simulink model "tank"  (R2015b)
settings: Solver=FixedStepDiscrete  StartTime=0.0  StopTime=inf  FixedStep=1e-3  RelTol=1e-3
libraries: sh_lib x74, nesl_utility x46, fl_lib x40, dspnetwork x33
(part 2 of 3)

== system tank/Virtual Gas Pipeline /The Gas Pipeline/Ball Valve2 ==
  Relief Valve Control : Inport
  Ball Valve : sh_lib/Valves/Flow Control Valves/Ball Valve  d_ball=8 in  d_orif=6 in  x_0=0 m  C_d=0.65  Re_cr=10  A_leak=1e-12 m^2
  Simulink-PS Converter : nesl_utility/Simulink-PS Converter  PhysicalDomain=network_engine_domain  SubClassName=ps_input  LeftPortType=input  RightPortType=output  PseudoPeriodic=off  Frequencies=[]  NoiseDistribution=none  NoiseParameters=[]  Unit=1  AffineConversion=off  InputFiltering=off  SimscapeFilterOrder=1  InputFilterTimeConstant=0.001  UdotUserProvided=1
  Inlet : PMIOPort  Port=1  Side=Left
  outlet : PMIOPort  Port=2  Side=Right
  wires:
  Relief Valve Control/1 -> Simulink-PS Converter/1
  connections:
  Simulink-PS Converter/RConn1 -- Ball Valve/LConn1
  Inlet/RConn1 -- Ball Valve/LConn2
  outlet/RConn1 -- Ball Valve/RConn1

== system tank/Virtual Gas Pipeline /The Gas Pipeline/Ball Valve3 ==
  Relief Valve Control : Inport
  Ball Valve : sh_lib/Valves/Flow Control Valves/Ball Valve  d_ball=8 in  d_orif=6 in  x_0=0 m  C_d=0.65  Re_cr=10  A_leak=1e-12 m^2
  Simulink-PS Converter : nesl_utility/Simulink-PS Converter  PhysicalDomain=network_engine_domain  SubClassName=ps_input  LeftPortType=input  RightPortType=output  PseudoPeriodic=off  Frequencies=[]  NoiseDistribution=none  NoiseParameters=[]  Unit=1  AffineConversion=off  InputFiltering=off  SimscapeFilterOrder=1  InputFilterTimeConstant=0.001  UdotUserProvided=1
  Inlet : PMIOPort  Port=1  Side=Left
  outlet : PMIOPort  Port=2  Side=Right
  wires:
  Relief Valve Control/1 -> Simulink-PS Converter/1
  connections:
  Simulink-PS Converter/RConn1 -- Ball Valve/LConn1
  Inlet/RConn1 -- Ball Valve/LConn2
  outlet/RConn1 -- Ball Valve/RConn1

== system tank/Virtual Gas Pipeline /The Gas Pipeline/Ball Valve4 ==
  valve : Inport
  Ball Valve : sh_lib/Valves/Flow Control Valves/Ball Valve  d_ball=18 in  d_orif=16 in  x_0=0 m  C_d=0.65  Re_cr=10  A_leak=1e-12 m^2
  Simulink-PS Converter : nesl_utility/Simulink-PS Converter  PhysicalDomain=network_engine_domain  SubClassName=ps_input  LeftPortType=input  RightPortType=output  PseudoPeriodic=off  Frequencies=[]  NoiseDistribution=none  NoiseParameters=[]  Unit=1  AffineConversion=off  InputFiltering=off  SimscapeFilterOrder=1  InputFilterTimeConstant=0.001  UdotUserProvided=1
  Inlet : PMIOPort  Port=1  Side=Left
  outlet : PMIOPort  Port=2  Side=Right
  wires:
  valve/1 -> Simulink-PS Converter/1
  connections:
  Simulink-PS Converter/RConn1 -- Ball Valve/LConn1
  Inlet/RConn1 -- Ball Valve/LConn2
  outlet/RConn1 -- Ball Valve/RConn1

== system tank/Virtual Gas Pipeline /The Gas Pipeline/Ball Valve5 ==
  valve : Inport
  Ball Valve : sh_lib/Valves/Flow Control Valves/Ball Valve  d_ball=18 in  d_orif=16 in  x_0=0 m  C_d=0.65  Re_cr=10  A_leak=1e-12 m^2
  Simulink-PS Converter : nesl_utility/Simulink-PS Converter  PhysicalDomain=network_engine_domain  SubClassName=ps_input  LeftPortType=input  RightPortType=output  PseudoPeriodic=off  Frequencies=[]  NoiseDistribution=none  NoiseParameters=[]  Unit=1  AffineConversion=off  InputFiltering=off  SimscapeFilterOrder=1  InputFilterTimeConstant=0.001  UdotUserProvided=1
  Inlet : PMIOPort  Port=1  Side=Left
  outlet : PMIOPort  Port=2  Side=Right
  wires:
  valve/1 -> Simulink-PS Converter/1
  connections:
  Simulink-PS Converter/RConn1 -- Ball Valve/LConn1
  Inlet/RConn1 -- Ball Valve/LConn2
  outlet/RConn1 -- Ball Valve/RConn1

== system tank/Virtual Gas Pipeline /The Gas Pipeline/Ball Valve6 ==
  valve : Inport
  Ball Valve : sh_lib/Valves/Flow Control Valves/Ball Valve  d_ball=8 in  d_orif=6 in  x_0=0 m  C_d=0.65  Re_cr=10  A_leak=1e-12 m^2
  Simulink-PS Converter : nesl_utility/Simulink-PS Converter  PhysicalDomain=network_engine_domain  SubClassName=ps_input  LeftPortType=input  RightPortType=output  PseudoPeriodic=off  Frequencies=[]  NoiseDistribution=none  NoiseParameters=[]  Unit=1  AffineConversion=off  InputFiltering=off  SimscapeFilterOrder=1  InputFilterTimeConstant=0.001  UdotUserProvided=1
  Inlet : PMIOPort  Port=1  Side=Left
  outlet : PMIOPort  Port=2  Side=Right
  wires:
  valve/1 -> Simulink-PS Converter/1
  connections:
  Simulink-PS Converter/RConn1 -- Ball Valve/LConn1
  Inlet/RConn1 -- Ball Valve/LConn2
  outlet/RConn1 -- Ball Valve/RConn1

== system tank/Virtual Gas Pipeline /The Gas Pipeline/Ball Valve7 ==
  valve : Inport
  Ball Valve : sh_lib/Valves/Flow Control Valves/Ball Valve  d_ball=8 in  d_orif=6 in  x_0=0 m  C_d=0.65  Re_cr=10  A_leak=1e-12 m^2
  Simulink-PS Converter : nesl_utility/Simulink-PS Converter  PhysicalDomain=network_engine_domain  SubClassName=ps_input  LeftPortType=input  RightPortType=output  PseudoPeriodic=off  Frequencies=[]  NoiseDistribution=none  NoiseParameters=[]  Unit=1  AffineConversion=off  InputFiltering=off  SimscapeFilterOrder=1  InputFilterTimeConstant=0.001  UdotUserProvided=1
  Inlet : PMIOPort  Port=1  Side=Left
  outlet : PMIOPort  Port=2  Side=Right
  wires:
  valve/1 -> Simulink-PS Converter/1
  connections:
  Simulink-PS Converter/RConn1 -- Ball Valve/LConn1
  Inlet/RConn1 -- Ball Valve/LConn2
  outlet/RConn1 -- Ball Valve/RConn1

== system tank/Virtual Gas Pipeline /The Gas Pipeline/Flow Measurement (KL//Hr) ==
  Constant : Constant  Value=3600
  Hydraulic Flow Rate Sensor : fl_lib/Hydraulic/Hydraulic Sensors/Hydraulic Flow Rate Sensor
  PS-Simulink Converter3 : nesl_utility/PS-Simulink Converter  PhysicalDomain=network_engine_domain  SubClassName=ps_output  LeftPortType=input  RightPortType=output  PseudoPeriodic=off  Frequencies=[]  Unit=m^3/s  AffineConversion=off
  Product : Product
  Inlet reference : PMIOPort  Port=1  Side=Left
  " Outlet Reference" : PMIOPort  Port=2  Side=Left
  Display out : Outport
  wires:
  Product/1 -> Display out/1
  Constant/1 -> Product/2
  PS-Simulink Converter3/1 -> Product/1
  connections:
  PS-Simulink Converter3/LConn1 -- Hydraulic Flow Rate Sensor/RConn1
  Hydraulic Flow Rate Sensor/RConn2 -- " Outlet Reference"/RConn1
  Hydraulic Flow Rate Sensor/LConn1 -- Inlet reference/RConn1

== system tank/Virtual Gas Pipeline /The Gas Pipeline/Flow Measurement (KL//Hr)1 ==
  Constant : Constant  Value=3600
  Hydraulic Flow Rate Sensor : fl_lib/Hydraulic/Hydraulic Sensors/Hydraulic Flow Rate Sensor
  PS-Simulink Converter3 : nesl_utility/PS-Simulink Converter  PhysicalDomain=network_engine_domain  SubClassName=ps_output  LeftPortType=input  RightPortType=output  PseudoPeriodic=off  Frequencies=[]  Unit=m^3/s  AffineConversion=off
  Product : Product
  Inlet reference : PMIOPort  Port=1  Side=Left
  " Outlet Reference" : PMIOPort  Port=2  Side=Left
  Display out : Outport
  wires:
  Product/1 -> Display out/1
  Constant/1 -> Product/2
  PS-Simulink Converter3/1 -> Product/1
  connections:
  PS-Simulink Converter3/LConn1 -- Hydraulic Flow Rate Sensor/RConn1
  Hydraulic Flow Rate Sensor/RConn2 -- " Outlet Reference"/RConn1
  Hydraulic Flow Rate Sensor/LConn1 -- Inlet reference/RConn1

== system tank/Virtual Gas Pipeline /The Gas Pipeline/Flow Measurement (KL//Hr)2 ==
  Constant : Constant  Value=3600
  Hydraulic Flow Rate Sensor : fl_lib/Hydraulic/Hydraulic Sensors/Hydraulic Flow Rate Sensor
  PS-Simulink Converter3 : nesl_utility/PS-Simulink Converter  PhysicalDomain=network_engine_domain  SubClassName=ps_output  LeftPortType=input  RightPortType=output  PseudoPeriodic=off  Frequencies=[]  Unit=m^3/s  AffineConversion=off
  Product : Product
  Inlet reference : PMIOPort  Port=1  Side=Left
  " Outlet Reference" : PMIOPort  Port=2  Side=Left
  Display out : Outport
  wires:
  Product/1 -> Display out/1
  Constant/1 -> Product/2
  PS-Simulink Converter3/1 -> Product/1
  connections:
  PS-Simulink Converter3/LConn1 -- Hydraulic Flow Rate Sensor/RConn1
  Hydraulic Flow Rate Sensor/RConn2 -- " Outlet Reference"/RConn1
  Hydraulic Flow Rate Sensor/LConn1 -- Inlet reference/RConn1

== system tank/Virtual Gas Pipeline /The Gas Pipeline/Flow Measurement (KL//Hr)3 ==
  Constant : Constant  Value=3600
  Hydraulic Flow Rate Sensor : fl_lib/Hydraulic/Hydraulic Sensors/Hydraulic Flow Rate Sensor
  PS-Simulink Converter3 : nesl_utility/PS-Simulink Converter  PhysicalDomain=network_engine_domain  SubClassName=ps_output  LeftPortType=input  RightPortType=output  PseudoPeriodic=off  Frequencies=[]  Unit=m^3/s  AffineConversion=off
  Product : Product
  Inlet reference : PMIOPort  Port=1  Side=Left
  " Outlet Reference" : PMIOPort  Port=2  Side=Left
  Display out : Outport
  wires:
  Product/1 -> Display out/1
  Constant/1 -> Product/2
  PS-Simulink Converter3/1 -> Product/1
  connections:
  PS-Simulink Converter3/LConn1 -- Hydraulic Flow Rate Sensor/RConn1
  Hydraulic Flow Rate Sensor/RConn2 -- " Outlet Reference"/RConn1
  Hydraulic Flow Rate Sensor/LConn1 -- Inlet reference/RConn1

== system tank/Virtual Gas Pipeline /The Gas Pipeline/Flow Measurement (KL//Hr)4 ==
  Constant : Constant  Value=3600
  Hydraulic Flow Rate Sensor : fl_lib/Hydraulic/Hydraulic Sensors/Hydraulic Flow Rate Sensor
  PS-Simulink Converter3 : nesl_utility/PS-Simulink Converter  PhysicalDomain=network_engine_domain  SubClassName=ps_output  LeftPortType=input  RightPortType=output  PseudoPeriodic=off  Frequencies=[]  Unit=m^3/s  AffineConversion=off
  Product : Product
  Inlet reference : PMIOPort  Port=1  Side=Left
  " Outlet Reference" : PMIOPort  Port=2  Side=Left
  Display out : Outport
  wires:
  Product/1 -> Display out/1
  Constant/1 -> Product/2
  PS-Simulink Converter3/1 -> Product/1
  connections:
  PS-Simulink Converter3/LConn1 -- Hydraulic Flow Rate Sensor/RConn1
  Hydraulic Flow Rate Sensor/RConn2 -- " Outlet Reference"/RConn1
  Hydraulic Flow Rate Sensor/LConn1 -- Inlet reference/RConn1

== system tank/Virtual Gas Pipeline /The Gas Pipeline/Flow Measurement (KL//Hr)5 ==
  Constant : Constant  Value=3600
  Hydraulic Flow Rate Sensor : fl_lib/Hydraulic/Hydraulic Sensors/Hydraulic Flow Rate Sensor
  PS-Simulink Converter3 : nesl_utility/PS-Simulink Converter  PhysicalDomain=network_engine_domain  SubClassName=ps_output  LeftPortType=input  RightPortType=output  PseudoPeriodic=off  Frequencies=[]  Unit=m^3/s  AffineConversion=off
  Product : Product
  Inlet reference : PMIOPort  Port=1  Side=Left
  " Outlet Reference" : PMIOPort  Port=2  Side=Left
  Display out : Outport
  wires:
  Product/1 -> Display out/1
  Constant/1 -> Product/2
  PS-Simulink Converter3/1 -> Product/1
  connections:
  PS-Simulink Converter3/LConn1 -- Hydraulic Flow Rate Sensor/RConn1
  Hydraulic Flow Rate Sensor/RConn2 -- " Outlet Reference"/RConn1
  Hydraulic Flow Rate Sensor/LConn1 -- Inlet reference/RConn1

== system tank/Virtual Gas Pipeline /The Gas Pipeline/Flow Measurement (KL//Hr)6 ==
  Constant : Constant  Value=3600
  Hydraulic Flow Rate Sensor : fl_lib/Hydraulic/Hydraulic Sensors/Hydraulic Flow Rate Sensor
  PS-Simulink Converter3 : nesl_utility/PS-Simulink Converter  PhysicalDomain=network_engine_domain  SubClassName=ps_output  LeftPortType=input  RightPortType=output  PseudoPeriodic=off  Frequencies=[]  Unit=m^3/s  AffineConversion=off
  Product : Product
  Inlet reference : PMIOPort  Port=1  Side=Left
  " Outlet Reference" : PMIOPort  Port=2  Side=Left
  Display out : Outport
  wires:
  Product/1 -> Display out/1
  Constant/1 -> Product/2
  PS-Simulink Converter3/1 -> Product/1
  connections:
  PS-Simulink Converter3/LConn1 -- Hydraulic Flow Rate Sensor/RConn1
  Hydraulic Flow Rate Sensor/RConn2 -- " Outlet Reference"/RConn1
  Hydraulic Flow Rate Sensor/LConn1 -- Inlet reference/RConn1

== system tank/Virtual Gas Pipeline /The Gas Pipeline/Flow Measurement (KL//Hr)7 ==
  Constant : Constant  Value=3600
  Hydraulic Flow Rate Sensor : fl_lib/Hydraulic/Hydraulic Sensors/Hydraulic Flow Rate Sensor
  PS-Simulink Converter3 : nesl_utility/PS-Simulink Converter  PhysicalDomain=network_engine_domain  SubClassName=ps_output  LeftPortType=input  RightPortType=output  PseudoPeriodic=off  Frequencies=[]  Unit=m^3/s  AffineConversion=off
  Product : Product
  Inlet reference : PMIOPort  Port=1  Side=Left
  " Outlet Reference" : PMIOPort  Port=2  Side=Left
  Display out : Outport
  wires:
  Product/1 -> Display out/1
  Constant/1 -> Product/2
  PS-Simulink Converter3/1 -> Product/1
  connections:
  PS-Simulink Converter3/LConn1 -- Hydraulic Flow Rate Sensor/RConn1
  Hydraulic Flow Rate Sensor/RConn2 -- " Outlet Reference"/RConn1
  Hydraulic Flow Rate Sensor/LConn1 -- Inlet reference/RConn1

== system tank/Virtual Gas Pipeline /The Gas Pipeline/Pressure Sensor ==
  Hydraulic Reference3 : fl_lib/Hydraulic/Hydraulic Elements/Hydraulic Reference
  Ideal Hydraulic Pressure Sensor3 : fl_lib/Hydraulic/Hydraulic Sensors/Hydraulic Pressure Sensor
  PS-Simulink Converter3 : nesl_utility/PS-Simulink Converter  PhysicalDomain=network_engine_domain  SubClassName=ps_output  LeftPortType=input  RightPortType=output  PseudoPeriodic=off  Frequencies=[]  Unit=Pa  AffineConversion=off
  Point : PMIOPort  Port=1  Side=Left
  " Display" : Outport
  wires:
  PS-Simulink Converter3/1 -> " Display"/1
  connections:
  Point/RConn1 -- Ideal Hydraulic Pressure Sensor3/LConn1
  Ideal Hydraulic Pressure Sensor3/RConn1 -- Hydraulic Reference3/LConn1
  Ideal Hydraulic Pressure Sensor3/RConn2 -- PS-Simulink Converter3/LConn1

== system tank/Virtual Gas Pipeline /The Gas Pipeline/Pressure Sensor1 ==
  Hydraulic Reference3 : fl_lib/Hydraulic/Hydraulic Elements/Hydraulic Reference
  Ideal Hydraulic Pressure Sensor3 : fl_lib/Hydraulic/Hydraulic Sensors/Hydraulic Pressure Sensor
  PS-Simulink Converter3 : nesl_utility/PS-Simulink Converter  PhysicalDomain=network_engine_domain  SubClassName=ps_output  LeftPortType=input  RightPortType=output  PseudoPeriodic=off  Frequencies=[]  Unit=Pa  AffineConversion=off
  Point : PMIOPort  Port=1  Side=Left
  " Display" : Outport
  wires:
  PS-Simulink Converter3/1 -> " Display"/1
  connections:
  Point/RConn1 -- Ideal Hydraulic Pressure Sensor3/LConn1
  Ideal Hydraulic Pressure Sensor3/RConn1 -- Hydraulic Reference3/LConn1
  Ideal Hydraulic Pressure Sensor3/RConn2 -- PS-Simulink Converter3/LConn1

== system tank/Virtual Gas Pipeline /The Gas Pipeline/Pressure Sensor2 ==
  Hydraulic Reference3 : fl_lib/Hydraulic/Hydraulic Elements/Hydraulic Reference
  Ideal Hydraulic Pressure Sensor3 : fl_lib/Hydraulic/Hydraulic Sensors/Hydraulic Pressure Sensor
  PS-Simulink Converter3 : nesl_utility/PS-Simulink Converter  PhysicalDomain=network_engine_domain  SubClassName=ps_output  LeftPortType=input  RightPortType=output  PseudoPeriodic=off  Frequencies=[]  Unit=Pa  AffineConversion=off
  Point : PMIOPort  Port=1  Side=Left
  " Display" : Outport
  wires:
  PS-Simulink Converter3/1 -> " Display"/1
  connections:
  Point/RConn1 -- Ideal Hydraulic Pressure Sensor3/LConn1
  Ideal Hydraulic Pressure Sensor3/RConn1 -- Hydraulic Reference3/LConn1
  Ideal Hydraulic Pressure Sensor3/RConn2 -- PS-Simulink Converter3/LConn1

== system tank/Virtual Gas Pipeline /The Gas Pipeline/Pressure Sensor3 ==
  Hydraulic Reference3 : fl_lib/Hydraulic/Hydraulic Elements/Hydraulic Reference
  Ideal Hydraulic Pressure Sensor3 : fl_lib/Hydraulic/Hydraulic Sensors/Hydraulic Pressure Sensor
  PS-Simulink Converter3 : nesl_utility/PS-Simulink Converter  PhysicalDomain=network_engine_domain  SubClassName=ps_output  LeftPortType=input  RightPortType=output  PseudoPeriodic=off  Frequencies=[]  Unit=Pa  AffineConversion=off
  Point : PMIOPort  Port=1  Side=Left
  " Display" : Outport
  wires:
  PS-Simulink Converter3/1 -> " Display"/1
  connections:
  Point/RConn1 -- Ideal Hydraulic Pressure Sensor3/LConn1
  Ideal Hydraulic Pressure Sensor3/RConn1 -- Hydraulic Reference3/LConn1
  Ideal Hydraulic Pressure Sensor3/RConn2 -- PS-Simulink Converter3/LConn1

== system tank/Virtual Gas Pipeline /The Gas Pipeline/Pressure Sensor4 ==
  Hydraulic Reference3 : fl_lib/Hydraulic/Hydraulic Elements/Hydraulic Reference
  Ideal Hydraulic Pressure Sensor3 : fl_lib/Hydraulic/Hydraulic Sensors/Hydraulic Pressure Sensor
  PS-Simulink Converter3 : nesl_utility/PS-Simulink Converter  PhysicalDomain=network_engine_domain  SubClassName=ps_output  LeftPortType=input  RightPortType=output  PseudoPeriodic=off  Frequencies=[]  Unit=Pa  AffineConversion=off
  Point : PMIOPort  Port=1  Side=Left
  " Display" : Outport
  wires:
  PS-Simulink Converter3/1 -> " Display"/1
  connections:
  Point/RConn1 -- Ideal Hydraulic Pressure Sensor3/LConn1
  Ideal Hydraulic Pressure Sensor3/RConn1 -- Hydraulic Reference3/LConn1
  Ideal Hydraulic Pressure Sensor3/RConn2 -- PS-Simulink Converter3/LConn1

== system tank/Virtual Gas Pipeline /The Gas Pipeline/Primary Pumping station (500 kl//hr) ==
  Pump 1 Control : Inport
  Fixed-Displacement Pump : sh_lib/Pumps and Motors/Fixed-Displacement Pump  D=.0027777777 m^3/rev  efficiency_vol=0.92  efficiency_tot=0.8  pr_nominal=8.5 bar  w_nominal=3000 rpm  visc_nominal=18 cSt  dens_nominal=900 kg/m^3  k_leak=1e-11 m^3/s/Pa  efficiency_mech=0.7
  Ideal Angular Velocity Source : fl_lib/Mechanical/Mechanical Sources/Ideal Angular Velocity Source
  Mechanical Rotational Reference : fl_lib/Mechanical/Rotational Elements/Mechanical Rotational Reference
  Simulink-PS Converter : nesl_utility/Simulink-PS Converter  PhysicalDomain=network_engine_domain  SubClassName=ps_input  LeftPortType=input  RightPortType=output  PseudoPeriodic=off  Frequencies=[]  NoiseDistribution=none  NoiseParameters=[]  Unit=1  AffineConversion=off  InputFiltering=off  SimscapeFilterOrder=1  InputFilterTimeConstant=0.001  UdotUserProvided=1
  Solver Configuration : nesl_utility/Solver Configuration  PhysicalDomain=network_engine_domain  SubClassName=solver  LeftPortType=input  RightPortType=generic  Accelerate=off  Tones=[]  Harmonics=[]  SimulateNoise=off  Profile=off  UseLocalSampling=off  EnableSwitchedLinearOptims=on  FrequencyDomain=off  UseCCode=off  RelTol=0.001  AbsTol=1e-06  MinStep=1e-09  ToWorkspace=off  RevertToSquareIcSolve=off  NumHomotopyIterations=100  PhasorMode=off  PhasorModeNumHarmonics=1  DoDC=on  ResidualTolerance=1  UseLocalSolver=on  LocalSolverChoice=NE_TRAPEZOIDAL_ADVANCER  LocalSolverSampleTime=0.001  DoFixedCost=on  MaxNonlinIter=12  MaxModeIter=2  LinearAlgebra=Full  DelaysMemoryBudget=1024  AutomaticFiltering=on  FilteringTimeConstant=0.001
  Switch1 : Switch  Threshold=1
  rpm : Constant  Value=3000
  rpm1 : Constant  Value=0
  Pump Outlet : PMIOPort  Port=1  Side=Right
  Pump Inlet : PMIOPort  Port=2  Side=Left
  wires:
  Pump 1 Control/1 -> Switch1/2
  rpm1/1 -> Switch1/3
  Switch1/1 -> Simulink-PS Converter/1
  rpm/1 -> Switch1/1
  connections:
  Mechanical Rotational Reference/LConn1 -- Ideal Angular Velocity Source/RConn2
  Simulink-PS Converter/RConn1 -- Ideal Angular Velocity Source/RConn1
  Pump Outlet/RConn1 -- Fixed-Displacement Pump/RConn1
  Fixed-Displacement Pump/LConn1 -- Solver Configuration/RConn1 -- Ideal Angular Velocity Source/LConn1
  Pump Inlet/RConn1 -- Fixed-Displacement Pump/RConn2

== system tank/Virtual Gas Pipeline /The Gas Pipeline/Recirculation valve ==
  valve : Inport
  Ball Valve : sh_lib/Valves/Flow Control Valves/Ball Valve  d_ball=18 in  d_orif=16 in  x_0=0 m  C_d=0.65  Re_cr=10  A_leak=1e-12 m^2
  Simulink-PS Converter : nesl_utility/Simulink-PS Converter  PhysicalDomain=network_engine_domain  SubClassName=ps_input  LeftPortType=input  RightPortType=output  PseudoPeriodic=off  Frequencies=[]  NoiseDistribution=none  NoiseParameters=[]  Unit=1  AffineConversion=off  InputFiltering=off  SimscapeFilterOrder=1  InputFilterTimeConstant=0.001  UdotUserProvided=1
  Inlet : PMIOPort  Port=1  Side=Left
  outlet : PMIOPort  Port=2  Side=Right
  wires:
  valve/1 -> Simulink-PS Converter/1
  connections:
  Simulink-PS Converter/RConn1 -- Ball Valve/LConn1
  Inlet/RConn1 -- Ball Valve/LConn2
  outlet/RConn1 -- Ball Valve/RConn1

== system tank/Virtual Gas Pipeline /The Gas Pipeline/Relief Valve 1  ==
  Relief Valve 1 Control : Inport
  Relief Valve 1 : sh_lib/Valves/Flow Control Valves/Ball Valve  d_ball=10 in  d_orif=8 in  x_0=0 m  C_d=0.65  Re_cr=10  A_leak=1e-12 m^2
  Simulink-PS Converter1 : nesl_utility/Simulink-PS Converter  PhysicalDomain=network_engine_domain  SubClassName=ps_input  LeftPortType=input  RightPortType=output  PseudoPeriodic=off  Frequencies=[]  NoiseDistribution=none  NoiseParameters=[]  Unit=1  AffineConversion=off  InputFiltering=off  SimscapeFilterOrder=1  InputFilterTimeConstant=0.001  UdotUserProvided=1
  Inlet : PMIOPort  Port=1  Side=Left
  Outlet : PMIOPort  Port=2  Side=Left
  wires:
  Relief Valve 1 Control/1 -> Simulink-PS Converter1/1
  connections:
  Outlet/RConn1 -- Relief Valve 1/RConn1
  Simulink-PS Converter1/RConn1 -- Relief Valve 1/LConn1
  Inlet/RConn1 -- Relief Valve 1/LConn2

== system tank/Virtual Gas Pipeline /The Gas Pipeline/Return line ==
  Hydraulic Pipeline4 : sh_lib/Pipelines/Hydraulic Pipeline  cs_type=1  d_in=16 in  area=1e-04 m^2  D_h=0.0112 m  s_factor=64  length=3000 m  length_ad=200 m  roughness=1.5e-05 m  Re_lam=2e+03  Re_turb=4e+03  wall_type=1  pr_r_coef=2e-12 m/Pa  time_const=0.01 s  k_sh=1.4  initial_pressure=0 Pa
  Sudden Area Change1 : sh_lib/Local Hydraulic Resistances/Sudden Area Change  small_diam=8 in  large_diam=16 in  mdl_type=1  kp_c=1  Re_vec="[  -4e+03 -3e+03 -2e+03 -1000 -500 -200 -100 -50 -40 -30 -20 -15 -10 10 20 30 40 50 100 200 500 1000 2e+03 4e+03 5e+03 1e+04 ]"  loss_coeff_vec="[  0.25 0.3 0.65 0.9 0.65 0.75 0.9 1.15 1.35 1.65 2.3 2.8 3.1 5 2.7 1.8 1.46 1.3 0.9 0.65 0.42 0.3 0.2 0.4 0.42 0.25 ]"  interp_method=2  extrap_method=2  Re_cr=110
  Return Inlet : PMIOPort  Port=1  Side=Left
  Return Outlet : PMIOPort  Port=2  Side=Right
  connections:
  Sudden Area Change1/RConn1 -- Hydraulic Pipeline4/LConn1
  Return Inlet/RConn1 -- Sudden Area Change1/LConn1
  Return Outlet/RConn1 -- Hydraulic Pipeline4/RConn1

== system tank/Virtual Gas Pipeline /The Gas Pipeline/Return line 1  ==
  Hydraulic Pipeline4 : sh_lib/Pipelines/Hydraulic Pipeline  cs_type=1  d_in=16 in  area=1e-04 m^2  D_h=0.0112 m  s_factor=64  length=3000 m  length_ad=200 m  roughness=1.5e-05 m  Re_lam=2e+03  Re_turb=4e+03  wall_type=1  pr_r_coef=2e-12 m/Pa  time_const=0.01 s  k_sh=1.4  initial_pressure=0 Pa
  Sudden Area Change1 : sh_lib/Local Hydraulic Resistances/Sudden Area Change  small_diam=8 in  large_diam=16 in  mdl_type=1  kp_c=1  Re_vec="[  -4e+03 -3e+03 -2e+03 -1000 -500 -200 -100 -50 -40 -30 -20 -15 -10 10 20 30 40 50 100 200 500 1000 2e+03 4e+03 5e+03 1e+04 ]"  loss_coeff_vec="[  0.25 0.3 0.65 0.9 0.65 0.75 0.9 1.15 1.35 1.65 2.3 2.8 3.1 5 2.7 1.8 1.46 1.3 0.9 0.65 0.42 0.3 0.2 0.4 0.42 0.25 ]"  interp_method=2  extrap_method=2  Re_cr=110
  Return Inlet : PMIOPort  Port=1  Side=Left
  Return Outlet : PMIOPort  Port=2  Side=Right
  connections:
  Sudden Area Change1/RConn1 -- Hydraulic Pipeline4/LConn1
  Return Inlet/RConn1 -- Sudden Area Change1/LConn1
  Return Outlet/RConn1 -- Hydraulic Pipeline4/RConn1

== system tank/Virtual Gas Pipeline /The Gas Pipeline/Return line1 ==
  Hydraulic Pipeline4 : sh_lib/Pipelines/Hydraulic Pipeline  cs_type=1  d_in=16 in  area=1e-04 m^2  D_h=0.0112 m  s_factor=64  length=3000 m  length_ad=200 m  roughness=1.5e-05 m  Re_lam=2e+03  Re_turb=4e+03  wall_type=1  pr_r_coef=2e-12 m/Pa  time_const=0.01 s  k_sh=1.4  initial_pressure=0 Pa
  Sudden Area Change1 : sh_lib/Local Hydraulic Resistances/Sudden Area Change  small_diam=8 in  large_diam=16 in  mdl_type=1  kp_c=1  Re_vec="[  -4e+03 -3e+03 -2e+03 -1000 -500 -200 -100 -50 -40 -30 -20 -15 -10 10 20 30 40 50 100 200 500 1000 2e+03 4e+03 5e+03 1e+04 ]"  loss_coeff_vec="[  0.25 0.3 0.65 0.9 0.65 0.75 0.9 1.15 1.35 1.65 2.3 2.8 3.1 5 2.7 1.8 1.46 1.3 0.9 0.65 0.42 0.3 0.2 0.4 0.42 0.25 ]"  interp_method=2  extrap_method=2  Re_cr=110
  Return Inlet : PMIOPort  Port=1  Side=Left
  Return Outlet : PMIOPort  Port=2  Side=Right
  connections:
  Sudden Area Change1/RConn1 -- Hydraulic Pipeline4/LConn1
  Return Inlet/RConn1 -- Sudden Area Change1/LConn1
  Return Outlet/RConn1 -- Hydraulic Pipeline4/RConn1

== system tank/Virtual Gas Pipeline /The Gas Pipeline/Return line2 ==
  Hydraulic Pipeline4 : sh_lib/Pipelines/Hydraulic Pipeline  cs_type=1  d_in=16 in  area=1e-04 m^2  D_h=0.0112 m  s_factor=64  length=3000 m  length_ad=200 m  roughness=1.5e-05 m  Re_lam=2e+03  Re_turb=4e+03  wall_type=1  pr_r_coef=2e-12 m/Pa  time_const=0.01 s  k_sh=1.4  initial_pressure=0 Pa
  Sudden Area Change1 : sh_lib/Local Hydraulic Resistances/Sudden Area Change  small_diam=8 in  large_diam=16 in  mdl_type=1  kp_c=1  Re_vec="[  -4e+03 -3e+03 -2e+03 -1000 -500 -200 -100 -50 -40 -30 -20 -15 -10 10 20 30 40 50 100 200 500 1000 2e+03 4e+03 5e+03 1e+04 ]"  loss_coeff_vec="[  0.25 0.3 0.65 0.9 0.65 0.75 0.9 1.15 1.35 1.65 2.3 2.8 3.1 5 2.7 1.8 1.46 1.3 0.9 0.65 0.42 0.3 0.2 0.4 0.42 0.25 ]"  interp_method=2  extrap_method=2  Re_cr=110
  Return Inlet : PMIOPort  Port=1  Side=Left
  Return Outlet : PMIOPort  Port=2  Side=Right
  connections:
  Sudden Area Change1/RConn1 -- Hydraulic Pipeline4/LConn1
  Return Inlet/RConn1 -- Sudden Area Change1/LConn1
  Return Outlet/RConn1 -- Hydraulic Pipeline4/RConn1

== system tank/Virtual Gas Pipeline /The Gas Pipeline/Return line3 ==
  Hydraulic Pipeline4 : sh_lib/Pipelines/Hydraulic Pipeline  cs_type=1  d_in=16 in  area=1e-04 m^2  D_h=0.0112 m  s_factor=64  length=3000 m  length_ad=200 m  roughness=1.5e-05 m  Re_lam=2e+03  Re_turb=4e+03  wall_type=1  pr_r_coef=2e-12 m/Pa  time_const=0.01 s  k_sh=1.4  initial_pressure=0 Pa
  Sudden Area Change1 : sh_lib/Local Hydraulic Resistances/Sudden Area Change  small_diam=8 in  large_diam=16 in  mdl_type=1  kp_c=1  Re_vec="[  -4e+03 -3e+03 -2e+03 -1000 -500 -200 -100 -50 -40 -30 -20 -15 -10 10 20 30 40 50 100 200 500 1000 2e+03 4e+03 5e+03 1e+04 ]"  loss_coeff_vec="[  0.25 0.3 0.65 0.9 0.65 0.75 0.9 1.15 1.35 1.65 2.3 2.8 3.1 5 2.7 1.8 1.46 1.3 0.9 0.65 0.42 0.3 0.2 0.4 0.42 0.25 ]"  interp_method=2  extrap_method=2  Re_cr=110
  Return Inlet : PMIOPort  Port=1  Side=Left
  Return Outlet : PMIOPort  Port=2  Side=Right
  connections:
  Sudden Area Change1/RConn1 -- Hydraulic Pipeline4/LConn1
  Return Inlet/RConn1 -- Sudden Area Change1/LConn1
  Return Outlet/RConn1 -- Hydraulic Pipeline4/RConn1

== system tank/Virtual Gas Pipeline /The Gas Pipeline/Source Return line body valve ==
  valve : Inport
  Ball Valve : sh_lib/Valves/Flow Control Valves/Ball Valve  d_ball=18 in  d_orif=16 in  x_0=0 m  C_d=0.65  Re_cr=10  A_leak=1e-12 m^2
  Simulink-PS Converter : nesl_utility/Simulink-PS Converter  PhysicalDomain=network_engine_domain  SubClassName=ps_input  LeftPortType=input  RightPortType=output  PseudoPeriodic=off  Frequencies=[]  NoiseDistribution=none  NoiseParameters=[]  Unit=1  AffineConversion=off  InputFiltering=off  SimscapeFilterOrder=1  InputFilterTimeConstant=0.001  UdotUserProvided=1
  Inlet : PMIOPort  Port=1  Side=Left
  outlet : PMIOPort  Port=2  Side=Right
  wires:
  valve/1 -> Simulink-PS Converter/1
  connections:
  Simulink-PS Converter/RConn1 -- Ball Valve/LConn1
  Inlet/RConn1 -- Ball Valve/LConn2
  outlet/RConn1 -- Ball Valve/RConn1

== system tank/Virtual Gas Pipeline /The Gas Pipeline/Source Return line body valve1 ==
  valve : Inport
  Ball Valve : sh_lib/Valves/Flow Control Valves/Ball Valve  d_ball=18 in  d_orif=16 in  x_0=0 m  C_d=0.65  Re_cr=10  A_leak=1e-12 m^2
  Simulink-PS Converter : nesl_utility/Simulink-PS Converter  PhysicalDomain=network_engine_domain  SubClassName=ps_input  LeftPortType=input  RightPortType=output  PseudoPeriodic=off  Frequencies=[]  NoiseDistribution=none  NoiseParameters=[]  Unit=1  AffineConversion=off  InputFiltering=off  SimscapeFilterOrder=1  InputFilterTimeConstant=0.001  UdotUserProvided=1
  Inlet : PMIOPort  Port=1  Side=Left
  outlet : PMIOPort  Port=2  Side=Right
  wires:
  valve/1 -> Simulink-PS Converter/1
  connections:
  Simulink-PS Converter/RConn1 -- Ball Valve/LConn1
  Inlet/RConn1 -- Ball Valve/LConn2
  outlet/RConn1 -- Ball Valve/RConn1

== system tank/Virtual Gas Pipeline /The Gas Pipeline/Source Tank Body Valve ==
  valve : Inport
  Ball Valve : sh_lib/Valves/Flow Control Valves/Ball Valve  d_ball=18 in  d_orif=16 in  x_0=0 m  C_d=0.65  Re_cr=10  A_leak=1e-12 m^2
  Simulink-PS Converter : nesl_utility/Simulink-PS Converter  PhysicalDomain=network_engine_domain  SubClassName=ps_input  LeftPortType=input  RightPortType=output  PseudoPeriodic=off  Frequencies=[]  NoiseDistribution=none  NoiseParameters=[]  Unit=1  AffineConversion=off  InputFiltering=off  SimscapeFilterOrder=1  InputFilterTimeConstant=0.001  UdotUserProvided=1
  Inlet : PMIOPort  Port=1  Side=Left
  outlet : PMIOPort  Port=2  Side=Right
  wires:
  valve/1 -> Simulink-PS Converter/1
  connections:
  Simulink-PS Converter/RConn1 -- Ball Valve/LConn1
  Inlet/RConn1 -- Ball Valve/LConn2
  outlet/RConn1 -- Ball Valve/RConn1

== system tank/Virtual Gas Pipeline /The Gas Pipeline/Source Tank Body Valve1 ==
  valve : Inport
  Ball Valve : sh_lib/Valves/Flow Control Valves/Ball Valve  d_ball=18 in  d_orif=16 in  x_0=0 m  C_d=0.65  Re_cr=10  A_leak=1e-12 m^2
  Simulink-PS Converter : nesl_utility/Simulink-PS Converter  PhysicalDomain=network_engine_domain  SubClassName=ps_input  LeftPortType=input  RightPortType=output  PseudoPeriodic=off  Frequencies=[]  NoiseDistribution=none  NoiseParameters=[]  Unit=1  AffineConversion=off  InputFiltering=off  SimscapeFilterOrder=1  InputFilterTimeConstant=0.001  UdotUserProvided=1
  Inlet : PMIOPort  Port=1  Side=Left
  outlet : PMIOPort  Port=2  Side=Right
  wires:
  valve/1 -> Simulink-PS Converter/1
  connections:
  Simulink-PS Converter/RConn1 -- Ball Valve/LConn1
  Inlet/RConn1 -- Ball Valve/LConn2
  outlet/RConn1 -- Ball Valve/RConn1

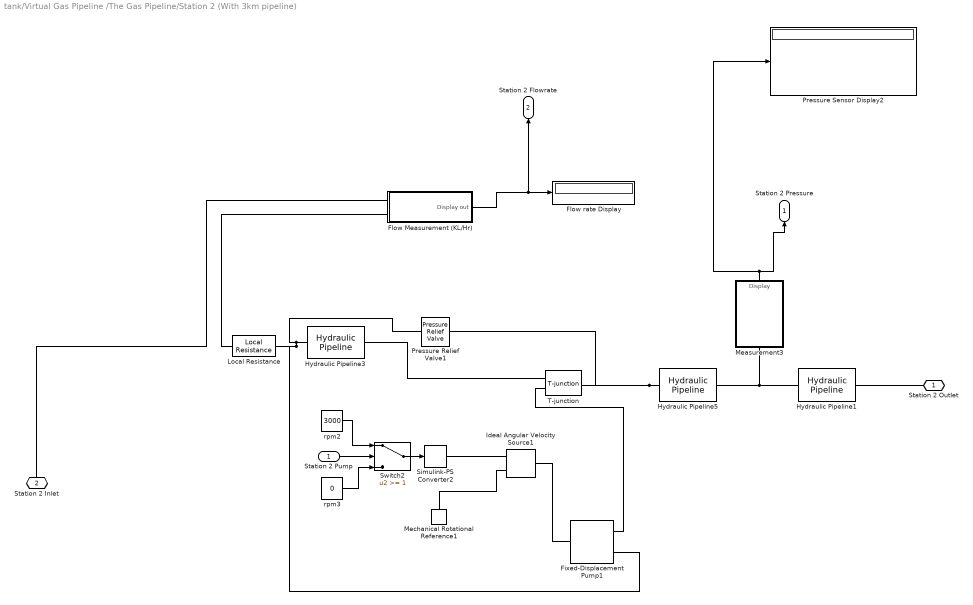
== system tank/Virtual Gas Pipeline /The Gas Pipeline/Station 2 (With 3km pipeline) ==
  Station 2 Pump : Inport
  Fixed-Displacement Pump1 : sh_lib/Pumps and Motors/Fixed-Displacement Pump  D=5e-4 m^3/rev  efficiency_vol=0.92  efficiency_tot=0.8  pr_nominal=8.5 bar  w_nominal=3000 rpm  visc_nominal=18 cSt  dens_nominal=900 kg/m^3  k_leak=1e-11 m^3/s/Pa  efficiency_mech=0.7
  Flow Measurement (KL/Hr) : Subsystem
  Flow rate Display : Display
  Hydraulic Pipeline1 : sh_lib/Pipelines/Hydraulic Pipeline  cs_type=1  d_in=16 in  area=1e-04 m^2  D_h=0.0112 m  s_factor=64  length=2900 m  length_ad=100 m  roughness=1.5e-3 m  Re_lam=2e+03  Re_turb=4e+03  wall_type=1  pr_r_coef=2e-12 m/Pa  time_const=0.01 s  k_sh=1.4  initial_pressure=0 Pa
  Hydraulic Pipeline3 : sh_lib/Pipelines/Hydraulic Pipeline  cs_type=1  d_in=16 in  area=1e-04 m^2  D_h=0.0112 m  s_factor=64  length=500 m  length_ad=500 m  roughness=1.5e-3 m  Re_lam=2e+03  Re_turb=4e+03  wall_type=1  pr_r_coef=2e-12 m/Pa  time_const=0.01 s  k_sh=1.4  initial_pressure=0 Pa
  Hydraulic Pipeline5 : sh_lib/Pipelines/Hydraulic Pipeline  cs_type=1  d_in=16 in  area=1e-04 m^2  D_h=0.0112 m  s_factor=64  length=100 m  length_ad=100 m  roughness=1.5e-3 m  Re_lam=2e+03  Re_turb=4e+03  wall_type=1  pr_r_coef=2e-12 m/Pa  time_const=0.01 s  k_sh=1.4  initial_pressure=0 Pa
  Ideal Angular Velocity Source1 : fl_lib/Mechanical/Mechanical Sources/Ideal Angular Velocity Source
  Local Resistance : sh_lib/Local Hydraulic Resistances/Local Resistance  area=25.12 in^2  mdl_type=1  kp_d=2  kp_r=2  Re_cr=150  Re_vec="[  -4e+03 -3e+03 -2e+03 -1000 -500 -200 -100 -50 -40 -30 -20 -15 -10 10 20 30 40 50 100 200 500 1000 2e+03 4e+03 5e+03 1e+04 ]"  loss_coeff_vec="[  0.25 0.3 0.65 0.9 0.65 0.75 0.9 1.15 1.35 1.65 2.3 2.8 3.1 5 2.7 1.8 1.46 1.3 0.9 0.65 0.42 0.3 0.2 0.4 0.42 0.25 ]"  interp_method=2  extrap_method=2  p_cr_d=1 Pa  p_cr_r=1 Pa  D_h=0.001 m
  Measurement3 : Subsystem
  Mechanical Rotational Reference1 : fl_lib/Mechanical/Rotational Elements/Mechanical Rotational Reference
  Pressure Relief Valve1 : sh_lib/Valves/Pressure Control Valves/Pressure Relief Valve  area_max=157 in^2  pres_set=150 psi  reg_range=5 psi  C_d=0.7  Re_cr=12  A_leak=1e-12 m^2  dynamic=0  tau=0.1 s  area_init=1e-12 m^2  gain=1 m^2/Pa  pr_max=55e5 Pa  f_cr=100 N
  Pressure Sensor Display2 : Display
  Simulink-PS Converter2 : nesl_utility/Simulink-PS Converter  PhysicalDomain=network_engine_domain  SubClassName=ps_input  LeftPortType=input  RightPortType=output  PseudoPeriodic=off  Frequencies=[]  NoiseDistribution=none  NoiseParameters=[]  Unit=1  AffineConversion=off  InputFiltering=off  SimscapeFilterOrder=1  InputFilterTimeConstant=0.001  UdotUserProvided=1
  Switch2 : Switch  Threshold=1
  T-junction : sh_lib/Local Hydraulic Resistances/T-junction  main_diam=16 in  branch_diam=16 in  kp_ab=1.12  kp_ba=1.12  kp_aa1=1.36  kp_a1a=1.65  kp_a1b=1.6  kp_ba1=1.8  Re_cr=120
  rpm2 : Constant  Value=3000
  rpm3 : Constant  Value=0
  Station 2 Outlet : PMIOPort  Port=1  Side=Right
  Station 2 Inlet : PMIOPort  Port=2  Side=Left
  Station 2 Pressure : Outport
  Station 2 Flowrate : Outport  Port=2
  wires:
  Switch2/1 -> Simulink-PS Converter2/1
  rpm2/1 -> Switch2/1
  Station 2 Pump/1 -> Switch2/2
  rpm3/1 -> Switch2/3
  Measurement3/1(Display) -> Pressure Sensor Display2/1, Station 2 Pressure/1
  Flow Measurement (KL/Hr)/1(Display out) -> Flow rate Display/1, Station 2 Flowrate/1
  connections:
  Station 2 Inlet/RConn1 -- Flow Measurement (KL/Hr)/LConn1
  Measurement3/LConn1 -- Hydraulic Pipeline1/LConn1 -- Hydraulic Pipeline5/RConn1
  Ideal Angular Velocity Source1/LConn1 -- Fixed-Displacement Pump1/LConn1
  Mechanical Rotational Reference1/LConn1 -- Ideal Angular Velocity Source1/RConn2
  Hydraulic Pipeline3/RConn1 -- T-junction/LConn1
  Hydraulic Pipeline3/LConn1 -- Fixed-Displacement Pump1/RConn2 -- Local Resistance/RConn1 -- Pressure Relief Valve1/RConn1
  Hydraulic Pipeline5/LConn1 -- Pressure Relief Valve1/LConn1 -- T-junction/RConn1
  Simulink-PS Converter2/RConn1 -- Ideal Angular Velocity Source1/RConn1
  T-junction/LConn2 -- Fixed-Displacement Pump1/RConn1
  Hydraulic Pipeline1/RConn1 -- Station 2 Outlet/RConn1
  Local Resistance/LConn1 -- Flow Measurement (KL/Hr)/LConn2

== system tank/Virtual Gas Pipeline /The Gas Pipeline/Station 2 inlet valve ==
  valve : Inport
  Ball Valve : sh_lib/Valves/Flow Control Valves/Ball Valve  d_ball=18 in  d_orif=16 in  x_0=0 m  C_d=0.65  Re_cr=10  A_leak=1e-12 m^2
  Simulink-PS Converter : nesl_utility/Simulink-PS Converter  PhysicalDomain=network_engine_domain  SubClassName=ps_input  LeftPortType=input  RightPortType=output  PseudoPeriodic=off  Frequencies=[]  NoiseDistribution=none  NoiseParameters=[]  Unit=1  AffineConversion=off  InputFiltering=off  SimscapeFilterOrder=1  InputFilterTimeConstant=0.001  UdotUserProvided=1
  Inlet : PMIOPort  Port=1  Side=Left
  outlet : PMIOPort  Port=2  Side=Right
  wires:
  valve/1 -> Simulink-PS Converter/1
  connections:
  Simulink-PS Converter/RConn1 -- Ball Valve/LConn1
  Inlet/RConn1 -- Ball Valve/LConn2
  outlet/RConn1 -- Ball Valve/RConn1

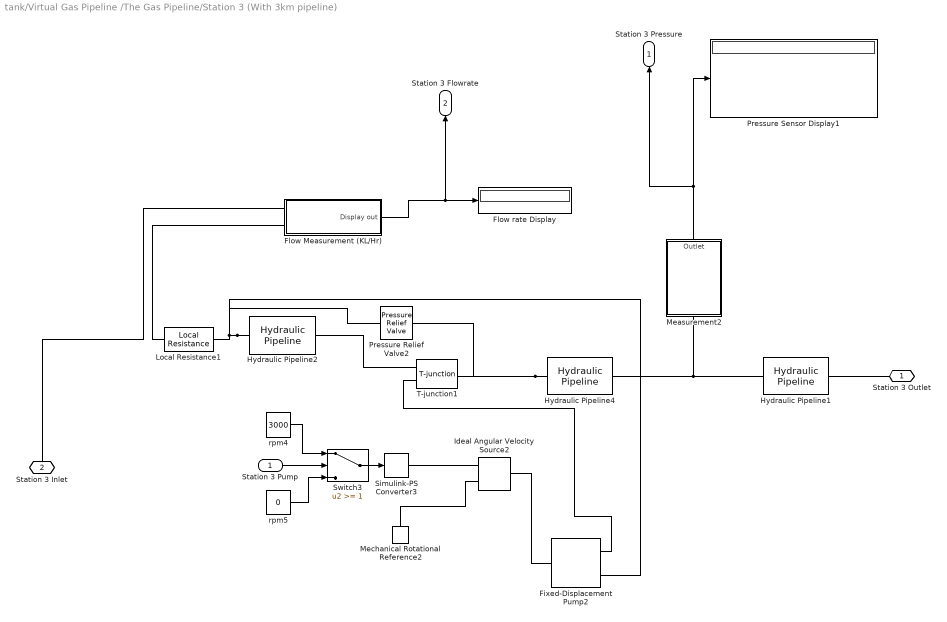
== system tank/Virtual Gas Pipeline /The Gas Pipeline/Station 3 (With 3km pipeline) ==
  Station 3 Pump : Inport
  Fixed-Displacement Pump2 : sh_lib/Pumps and Motors/Fixed-Displacement Pump  D=5e-4 m^3/rev  efficiency_vol=0.92  efficiency_tot=0.8  pr_nominal=8.5 bar  w_nominal=3000 rpm  visc_nominal=18 cSt  dens_nominal=900 kg/m^3  k_leak=1e-11 m^3/s/Pa  efficiency_mech=0.7
  Flow Measurement (KL/Hr) : Subsystem
  Flow rate Display : Display
  Hydraulic Pipeline1 : sh_lib/Pipelines/Hydraulic Pipeline  cs_type=1  d_in=16 in  area=1e-04 m^2  D_h=0.0112 m  s_factor=64  length=2900 m  length_ad=100 m  roughness=1.5e-3 m  Re_lam=2e+03  Re_turb=4e+03  wall_type=1  pr_r_coef=2e-12 m/Pa  time_const=0.01 s  k_sh=1.4  initial_pressure=0 Pa
  Hydraulic Pipeline2 : sh_lib/Pipelines/Hydraulic Pipeline  cs_type=1  d_in=16 in  area=1e-04 m^2  D_h=0.0112 m  s_factor=64  length=500 m  length_ad=500 m  roughness=1.5e-3 m  Re_lam=2e+03  Re_turb=4e+03  wall_type=1  pr_r_coef=2e-12 m/Pa  time_const=0.01 s  k_sh=1.4  initial_pressure=0 Pa
  Hydraulic Pipeline4 : sh_lib/Pipelines/Hydraulic Pipeline  cs_type=1  d_in=16 in  area=1e-04 m^2  D_h=0.0112 m  s_factor=64  length=100 m  length_ad=100 m  roughness=1.5e-3 m  Re_lam=2e+03  Re_turb=4e+03  wall_type=1  pr_r_coef=2e-12 m/Pa  time_const=0.01 s  k_sh=1.4  initial_pressure=0 Pa
  Ideal Angular Velocity Source2 : fl_lib/Mechanical/Mechanical Sources/Ideal Angular Velocity Source
  Local Resistance1 : sh_lib/Local Hydraulic Resistances/Local Resistance  area=25.12 in^2  mdl_type=1  kp_d=2  kp_r=2  Re_cr=150  Re_vec="[  -4e+03 -3e+03 -2e+03 -1000 -500 -200 -100 -50 -40 -30 -20 -15 -10 10 20 30 40 50 100 200 500 1000 2e+03 4e+03 5e+03 1e+04 ]"  loss_coeff_vec="[  0.25 0.3 0.65 0.9 0.65 0.75 0.9 1.15 1.35 1.65 2.3 2.8 3.1 5 2.7 1.8 1.46 1.3 0.9 0.65 0.42 0.3 0.2 0.4 0.42 0.25 ]"  interp_method=2  extrap_method=2  p_cr_d=1 Pa  p_cr_r=1 Pa  D_h=0.001 m
  Measurement2 : Subsystem
  Mechanical Rotational Reference2 : fl_lib/Mechanical/Rotational Elements/Mechanical Rotational Reference
  Pressure Relief Valve2 : sh_lib/Valves/Pressure Control Valves/Pressure Relief Valve  area_max=157 in^2  pres_set=150 psi  reg_range=5 psi  C_d=0.7  Re_cr=12  A_leak=1e-12 m^2  dynamic=0  tau=0.1 s  area_init=1e-12 m^2  gain=1 m^2/Pa  pr_max=55e5 Pa  f_cr=100 N
  Pressure Sensor Display1 : Display
  Simulink-PS Converter3 : nesl_utility/Simulink-PS Converter  PhysicalDomain=network_engine_domain  SubClassName=ps_input  LeftPortType=input  RightPortType=output  PseudoPeriodic=off  Frequencies=[]  NoiseDistribution=none  NoiseParameters=[]  Unit=1  AffineConversion=off  InputFiltering=off  SimscapeFilterOrder=1  InputFilterTimeConstant=0.001  UdotUserProvided=1
  Switch3 : Switch  Threshold=1
  T-junction1 : sh_lib/Local Hydraulic Resistances/T-junction  main_diam=16 in  branch_diam=16 in  kp_ab=1.12  kp_ba=1.12  kp_aa1=1.36  kp_a1a=1.65  kp_a1b=1.6  kp_ba1=1.8  Re_cr=120
  rpm4 : Constant  Value=3000
  rpm5 : Constant  Value=0
  Station 3 Outlet : PMIOPort  Port=1  Side=Right
  Station 3 Inlet : PMIOPort  Port=2  Side=Left
  Station 3 Pressure : Outport
  Station 3 Flowrate : Outport  Port=2
  wires:
  rpm4/1 -> Switch3/1
  Switch3/1 -> Simulink-PS Converter3/1
  rpm5/1 -> Switch3/3
  Station 3 Pump/1 -> Switch3/2
  Measurement2/1(Outlet) -> Pressure Sensor Display1/1, Station 3 Pressure/1
  Flow Measurement (KL/Hr)/1(Display out) -> Flow rate Display/1, Station 3 Flowrate/1
  connections:
  T-junction1/LConn2 -- Fixed-Displacement Pump2/RConn1
  Mechanical Rotational Reference2/LConn1 -- Ideal Angular Velocity Source2/RConn2
  Ideal Angular Velocity Source2/LConn1 -- Fixed-Displacement Pump2/LConn1
  Simulink-PS Converter3/RConn1 -- Ideal Angular Velocity Source2/RConn1
  Measurement2/LConn1 -- Hydraulic Pipeline4/RConn1 -- Hydraulic Pipeline1/LConn1
  Hydraulic Pipeline2/RConn1 -- T-junction1/LConn1
  Hydraulic Pipeline2/LConn1 -- Local Resistance1/RConn1 -- Pressure Relief Valve2/RConn1 -- Fixed-Displacement Pump2/RConn2
  Hydraulic Pipeline4/LConn1 -- Pressure Relief Valve2/LConn1 -- T-junction1/RConn1
  Station 3 Inlet/RConn1 -- Flow Measurement (KL/Hr)/LConn1
  Hydraulic Pipeline1/RConn1 -- Station 3 Outlet/RConn1
  Flow Measurement (KL/Hr)/LConn2 -- Local Resistance1/LConn1

== system tank/Virtual Gas Pipeline /The Gas Pipeline/Station 3 inlet valve ==
  valve : Inport
  Ball Valve : sh_lib/Valves/Flow Control Valves/Ball Valve  d_ball=18 in  d_orif=16 in  x_0=0 m  C_d=0.65  Re_cr=10  A_leak=1e-12 m^2
  Simulink-PS Converter : nesl_utility/Simulink-PS Converter  PhysicalDomain=network_engine_domain  SubClassName=ps_input  LeftPortType=input  RightPortType=output  PseudoPeriodic=off  Frequencies=[]  NoiseDistribution=none  NoiseParameters=[]  Unit=1  AffineConversion=off  InputFiltering=off  SimscapeFilterOrder=1  InputFilterTimeConstant=0.001  UdotUserProvided=1
  Inlet : PMIOPort  Port=1  Side=Left
  outlet : PMIOPort  Port=2  Side=Right
  wires:
  valve/1 -> Simulink-PS Converter/1
  connections:
  Simulink-PS Converter/RConn1 -- Ball Valve/LConn1
  Inlet/RConn1 -- Ball Valve/LConn2
  outlet/RConn1 -- Ball Valve/RConn1

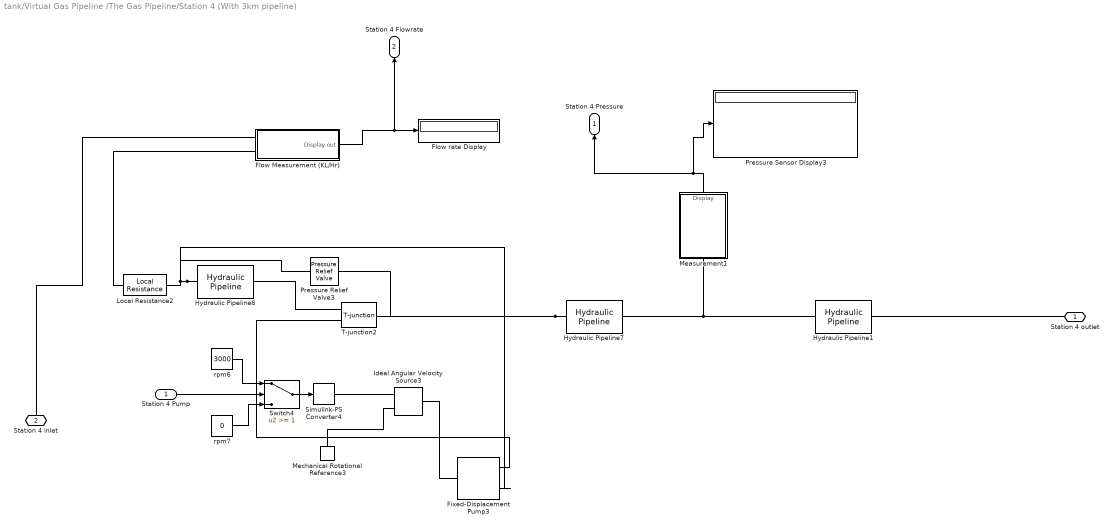
== system tank/Virtual Gas Pipeline /The Gas Pipeline/Station 4 (With 3km pipeline) ==
  "Station 4 Pump " : Inport
  Fixed-Displacement Pump3 : sh_lib/Pumps and Motors/Fixed-Displacement Pump  D=5e-4 m^3/rev  efficiency_vol=0.92  efficiency_tot=0.8  pr_nominal=8.5 bar  w_nominal=3000 rpm  visc_nominal=18 cSt  dens_nominal=900 kg/m^3  k_leak=1e-11 m^3/s/Pa  efficiency_mech=0.7
  Flow Measurement (KL/Hr) : Subsystem
  Flow rate Display : Display
  Hydraulic Pipeline1 : sh_lib/Pipelines/Hydraulic Pipeline  cs_type=1  d_in=16 in  area=1e-04 m^2  D_h=0.0112 m  s_factor=64  length=2900 m  length_ad=100 m  roughness=1.5e-3 m  Re_lam=2e+03  Re_turb=4e+03  wall_type=1  pr_r_coef=2e-12 m/Pa  time_const=0.01 s  k_sh=1.4  initial_pressure=0 Pa
  Hydraulic Pipeline6 : sh_lib/Pipelines/Hydraulic Pipeline  cs_type=1  d_in=16 in  area=1e-04 m^2  D_h=0.0112 m  s_factor=64  length=500 m  length_ad=500 m  roughness=1.5e-3 m  Re_lam=2e+03  Re_turb=4e+03  wall_type=1  pr_r_coef=2e-12 m/Pa  time_const=0.01 s  k_sh=1.4  initial_pressure=0 Pa
  Hydraulic Pipeline7 : sh_lib/Pipelines/Hydraulic Pipeline  cs_type=1  d_in=16 in  area=1e-04 m^2  D_h=0.0112 m  s_factor=64  length=100 m  length_ad=100 m  roughness=1.5e-3 m  Re_lam=2e+03  Re_turb=4e+03  wall_type=1  pr_r_coef=2e-12 m/Pa  time_const=0.01 s  k_sh=1.4  initial_pressure=0 Pa
  Ideal Angular Velocity Source3 : fl_lib/Mechanical/Mechanical Sources/Ideal Angular Velocity Source
  Local Resistance2 : sh_lib/Local Hydraulic Resistances/Local Resistance  area=25.12 in^2  mdl_type=1  kp_d=2  kp_r=2  Re_cr=150  Re_vec="[  -4e+03 -3e+03 -2e+03 -1000 -500 -200 -100 -50 -40 -30 -20 -15 -10 10 20 30 40 50 100 200 500 1000 2e+03 4e+03 5e+03 1e+04 ]"  loss_coeff_vec="[  0.25 0.3 0.65 0.9 0.65 0.75 0.9 1.15 1.35 1.65 2.3 2.8 3.1 5 2.7 1.8 1.46 1.3 0.9 0.65 0.42 0.3 0.2 0.4 0.42 0.25 ]"  interp_method=2  extrap_method=2  p_cr_d=1 Pa  p_cr_r=1 Pa  D_h=0.001 m
  Measurement1 : Subsystem
  Mechanical Rotational Reference3 : fl_lib/Mechanical/Rotational Elements/Mechanical Rotational Reference
  Pressure Relief Valve3 : sh_lib/Valves/Pressure Control Valves/Pressure Relief Valve  area_max=157 in^2  pres_set=150 psi  reg_range=5 psi  C_d=0.7  Re_cr=12  A_leak=1e-12 m^2  dynamic=0  tau=0.1 s  area_init=1e-12 m^2  gain=1 m^2/Pa  pr_max=55e5 Pa  f_cr=100 N
  Pressure Sensor Display3 : Display
  Simulink-PS Converter4 : nesl_utility/Simulink-PS Converter  PhysicalDomain=network_engine_domain  SubClassName=ps_input  LeftPortType=input  RightPortType=output  PseudoPeriodic=off  Frequencies=[]  NoiseDistribution=none  NoiseParameters=[]  Unit=1  AffineConversion=off  InputFiltering=off  SimscapeFilterOrder=1  InputFilterTimeConstant=0.001  UdotUserProvided=1
  Switch4 : Switch  Threshold=1
  T-junction2 : sh_lib/Local Hydraulic Resistances/T-junction  main_diam=16 in  branch_diam=16 in  kp_ab=1.12  kp_ba=1.12  kp_aa1=1.36  kp_a1a=1.65  kp_a1b=1.6  kp_ba1=1.8  Re_cr=120
  rpm6 : Constant  Value=3000
  rpm7 : Constant  Value=0
  Station 4 outlet : PMIOPort  Port=1  Side=Right
  Station 4 inlet : PMIOPort  Port=2  Side=Left
  Station 4 Pressure : Outport
  Station 4 Flowrate : Outport  Port=2
  wires:
  Switch4/1 -> Simulink-PS Converter4/1
  rpm6/1 -> Switch4/1
  "Station 4 Pump "/1 -> Switch4/2
  rpm7/1 -> Switch4/3
  Measurement1/1(Display) -> Pressure Sensor Display3/1, Station 4 Pressure/1
  Flow Measurement (KL/Hr)/1(Display out) -> Station 4 Flowrate/1, Flow rate Display/1
  connections:
  T-junction2/LConn2 -- Fixed-Displacement Pump3/RConn1
  Mechanical Rotational Reference3/LConn1 -- Ideal Angular Velocity Source3/RConn2
  Simulink-PS Converter4/RConn1 -- Ideal Angular Velocity Source3/RConn1
  Hydraulic Pipeline6/LConn1 -- Local Resistance2/RConn1 -- Pressure Relief Valve3/RConn1 -- Fixed-Displacement Pump3/RConn2
  Hydraulic Pipeline7/LConn1 -- Pressure Relief Valve3/LConn1 -- T-junction2/RConn1
  Hydraulic Pipeline6/RConn1 -- T-junction2/LConn1
  Measurement1/LConn1 -- Hydraulic Pipeline7/RConn1 -- Hydraulic Pipeline1/LConn1
  Ideal Angular Velocity Source3/LConn1 -- Fixed-Displacement Pump3/LConn1
  Station 4 inlet/RConn1 -- Flow Measurement (KL/Hr)/LConn1
  Hydraulic Pipeline1/RConn1 -- Station 4 outlet/RConn1
  Flow Measurement (KL/Hr)/LConn2 -- Local Resistance2/LConn1

== system tank/Virtual Gas Pipeline /The Gas Pipeline/Station 4 inlet valve ==
  valve : Inport
  Ball Valve : sh_lib/Valves/Flow Control Valves/Ball Valve  d_ball=18 in  d_orif=16 in  x_0=0 m  C_d=0.65  Re_cr=10  A_leak=1e-12 m^2
  Simulink-PS Converter : nesl_utility/Simulink-PS Converter  PhysicalDomain=network_engine_domain  SubClassName=ps_input  LeftPortType=input  RightPortType=output  PseudoPeriodic=off  Frequencies=[]  NoiseDistribution=none  NoiseParameters=[]  Unit=1  AffineConversion=off  InputFiltering=off  SimscapeFilterOrder=1  InputFilterTimeConstant=0.001  UdotUserProvided=1
  Inlet : PMIOPort  Port=1  Side=Left
  outlet : PMIOPort  Port=2  Side=Right
  wires:
  valve/1 -> Simulink-PS Converter/1
  connections:
  Simulink-PS Converter/RConn1 -- Ball Valve/LConn1
  Inlet/RConn1 -- Ball Valve/LConn2
  outlet/RConn1 -- Ball Valve/RConn1

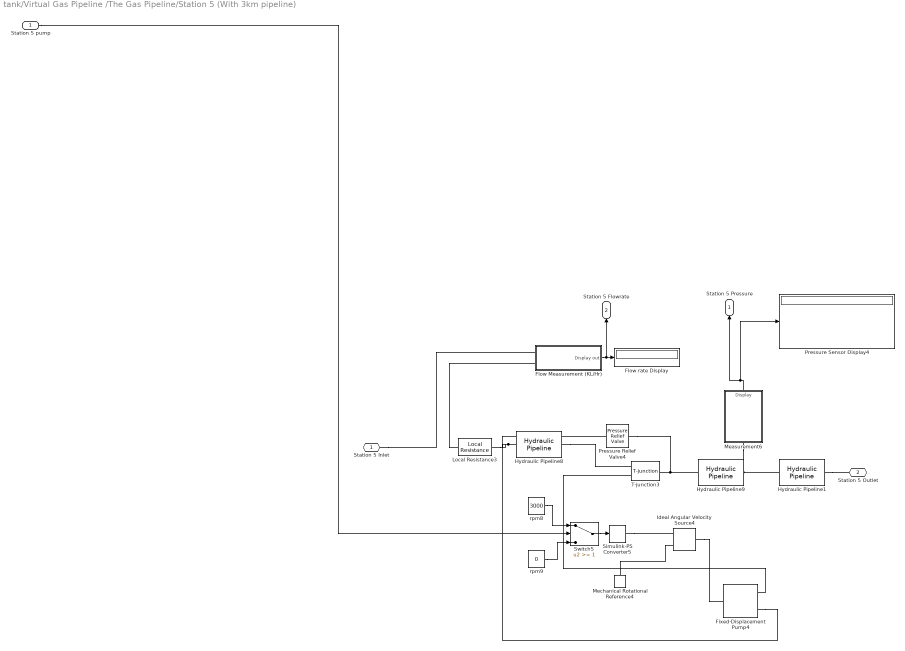
== system tank/Virtual Gas Pipeline /The Gas Pipeline/Station 5 (With 3km pipeline) ==
  Station 5 pump : Inport
  Fixed-Displacement Pump4 : sh_lib/Pumps and Motors/Fixed-Displacement Pump  D=5e-4 m^3/rev  efficiency_vol=0.92  efficiency_tot=0.8  pr_nominal=8.5 bar  w_nominal=3000 rpm  visc_nominal=18 cSt  dens_nominal=900 kg/m^3  k_leak=1e-11 m^3/s/Pa  efficiency_mech=0.7
  Flow Measurement (KL/Hr) : Subsystem
  Flow rate Display : Display
  Hydraulic Pipeline1 : sh_lib/Pipelines/Hydraulic Pipeline  cs_type=1  d_in=16 in  area=1e-04 m^2  D_h=0.0112 m  s_factor=64  length=2900 m  length_ad=100 m  roughness=1.5e-3 m  Re_lam=2e+03  Re_turb=4e+03  wall_type=1  pr_r_coef=2e-12 m/Pa  time_const=0.01 s  k_sh=1.4  initial_pressure=0 Pa
  Hydraulic Pipeline8 : sh_lib/Pipelines/Hydraulic Pipeline  cs_type=1  d_in=16 in  area=1e-04 m^2  D_h=0.0112 m  s_factor=64  length=500 m  length_ad=500 m  roughness=1.5e-3 m  Re_lam=2e+03  Re_turb=4e+03  wall_type=1  pr_r_coef=2e-12 m/Pa  time_const=0.01 s  k_sh=1.4  initial_pressure=0 Pa
  Hydraulic Pipeline9 : sh_lib/Pipelines/Hydraulic Pipeline  cs_type=1  d_in=16 in  area=1e-04 m^2  D_h=0.0112 m  s_factor=64  length=100 m  length_ad=100 m  roughness=1.5e-3 m  Re_lam=2e+03  Re_turb=4e+03  wall_type=1  pr_r_coef=2e-12 m/Pa  time_const=0.01 s  k_sh=1.4  initial_pressure=0 Pa
  Ideal Angular Velocity Source4 : fl_lib/Mechanical/Mechanical Sources/Ideal Angular Velocity Source
  Local Resistance3 : sh_lib/Local Hydraulic Resistances/Local Resistance  area=25.12 in^2  mdl_type=1  kp_d=2  kp_r=2  Re_cr=150  Re_vec="[  -4e+03 -3e+03 -2e+03 -1000 -500 -200 -100 -50 -40 -30 -20 -15 -10 10 20 30 40 50 100 200 500 1000 2e+03 4e+03 5e+03 1e+04 ]"  loss_coeff_vec="[  0.25 0.3 0.65 0.9 0.65 0.75 0.9 1.15 1.35 1.65 2.3 2.8 3.1 5 2.7 1.8 1.46 1.3 0.9 0.65 0.42 0.3 0.2 0.4 0.42 0.25 ]"  interp_method=2  extrap_method=2  p_cr_d=1 Pa  p_cr_r=1 Pa  D_h=0.001 m
  Measurement6 : Subsystem
  Mechanical Rotational Reference4 : fl_lib/Mechanical/Rotational Elements/Mechanical Rotational Reference
  Pressure Relief Valve4 : sh_lib/Valves/Pressure Control Valves/Pressure Relief Valve  area_max=157 in^2  pres_set=150 psi  reg_range=5 psi  C_d=0.7  Re_cr=12  A_leak=1e-12 m^2  dynamic=0  tau=0.1 s  area_init=1e-12 m^2  gain=1 m^2/Pa  pr_max=55e5 Pa  f_cr=100 N
  Pressure Sensor Display4 : Display
  Simulink-PS Converter5 : nesl_utility/Simulink-PS Converter  PhysicalDomain=network_engine_domain  SubClassName=ps_input  LeftPortType=input  RightPortType=output  PseudoPeriodic=off  Frequencies=[]  NoiseDistribution=none  NoiseParameters=[]  Unit=1  AffineConversion=off  InputFiltering=off  SimscapeFilterOrder=1  InputFilterTimeConstant=0.001  UdotUserProvided=1
  Switch5 : Switch  Threshold=1
  T-junction3 : sh_lib/Local Hydraulic Resistances/T-junction  main_diam=16 in  branch_diam=16 in  kp_ab=1.12  kp_ba=1.12  kp_aa1=1.36  kp_a1a=1.65  kp_a1b=1.6  kp_ba1=1.8  Re_cr=120
  rpm8 : Constant  Value=3000
  rpm9 : Constant  Value=0
  Station 5 Inlet : PMIOPort  Port=1  Side=Left
  Station 5 Outlet : PMIOPort  Port=2  Side=Right
  Station 5 Pressure : Outport
  Station 5 Flowrate : Outport  Port=2
  wires:
  rpm9/1 -> Switch5/3
  Switch5/1 -> Simulink-PS Converter5/1
  rpm8/1 -> Switch5/1
  Station 5 pump/1 -> Switch5/2
  Measurement6/1(Display) -> Pressure Sensor Display4/1, Station 5 Pressure/1
  Flow Measurement (KL/Hr)/1(Display out) -> Station 5 Flowrate/1, Flow rate Display/1
  connections:
  Simulink-PS Converter5/RConn1 -- Ideal Angular Velocity Source4/RConn1
  T-junction3/LConn2 -- Fixed-Displacement Pump4/RConn1
  Hydraulic Pipeline8/RConn1 -- T-junction3/LConn1
  Hydraulic Pipeline8/LConn1 -- Local Resistance3/RConn1 -- Pressure Relief Valve4/RConn1 -- Fixed-Displacement Pump4/RConn2
  Mechanical Rotational Reference4/LConn1 -- Ideal Angular Velocity Source4/RConn2
  Ideal Angular Velocity Source4/LConn1 -- Fixed-Displacement Pump4/LConn1
  Station 5 Inlet/RConn1 -- Flow Measurement (KL/Hr)/LConn1
  Hydraulic Pipeline1/RConn1 -- Station 5 Outlet/RConn1
  Hydraulic Pipeline1/LConn1 -- Hydraulic Pipeline9/RConn1 -- Measurement6/LConn1
  Pressure Relief Valve4/LConn1 -- Hydraulic Pipeline9/LConn1 -- T-junction3/RConn1
  Flow Measurement (KL/Hr)/LConn2 -- Local Resistance3/LConn1
